simulink model "prop_control_ALK_Assignment"  (R2020b)
settings: Solver=VariableStepAuto  StartTime=0.0  StopTime=3  RelTol=1e-3
settings Model: Creator=mario  LastModifiedBy=joconnor
settings DataIOCC: ReturnWorkspaceOutputs=off
settings DebuggingCC: ArithmeticOperatorsInVariantConditions=warning
settings SFSimCC: CustomCodeUndefinedFunction=UseInterfaceOnly

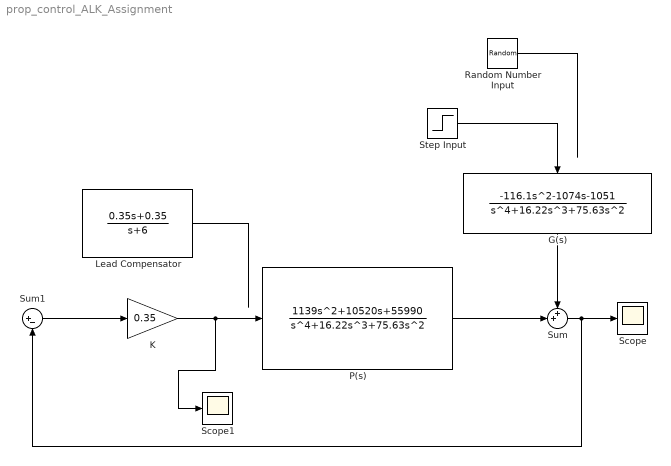
== system prop_control_ALK_Assignment ==
  G(s) : TransferFcn  Numerator=[-116.1 -1074 -1051]  Denominator=[1 16.22 75.63 0 0]
  K : Gain  Gain=0.35
  Lead Compensator : TransferFcn  Numerator=[0.35 0.35]  Denominator=[1 6]
  P(s) : TransferFcn  Numerator=[1139 10520 55990]  Denominator=[1 16.22 75.63 0 0]
  Random Number Input : RandomNumber  Variance=0.02723  Seed=1  SampleTime=6
  Scope : Scope
  Scope1 : Scope
  Step Input : Step  Time=0.5  After=0.02723  SampleTime=0
  Sum : Sum  Inputs=++|
  Sum1 : Sum  Inputs=|+-
  wires:
  G(s)/1 -> Sum/1
  P(s)/1 -> Sum/2
  K/1 -> Scope1/1, P(s)/1
  Sum/1 -> Scope/1, Sum1/2
  Random Number Input/1 -> ?
  Step Input/1 -> G(s)/1
  Sum1/1 -> K/1
  Lead Compensator/1 -> ?
